simulink model "masspringdamper"  (R2020a)
settings: Solver=VariableStepAuto  StartTime=0.0  StopTime=50  RelTol=1e-3
values from neighbouring files (symbols this model uses):
  b = 20    [systemparameter.m]
  F = 15    [systemparameter.m]
  k = 10    [systemparameter.m]
  M = 100    [systemparameter.m]
settings Model: Creator=diogo  LastModifiedBy=diogo

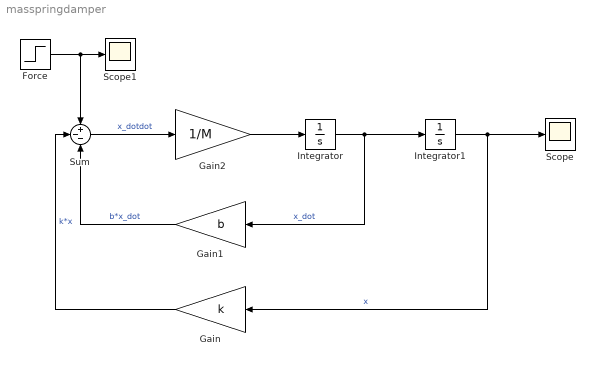
== system masspringdamper ==
  Force : Step  After=F  SampleTime=0
  Gain : Gain  Gain=k
  Gain1 : Gain  Gain=b
  Gain2 : Gain  Gain=1/M
  Integrator : Integrator
  Integrator1 : Integrator
  Scope : Scope
  Scope1 : Scope
  Sum : Sum  Inputs=+--
  wires:
  Integrator1/1 -> Scope/1, Gain/1  "x"
  Integrator/1 -> Gain1/1, Integrator1/1  "x_dot"
  Sum/1 -> Gain2/1  "x_dotdot"
  Force/1 -> Scope1/1, Sum/1
  Gain1/1 -> Sum/3  "b*x_dot"
  Gain/1 -> Sum/2  "k*x"
  Gain2/1 -> Integrator/1
